simulink model "Ackerman Model For Simulation"  (R2020b)
settings: Solver=ode4  StartTime=0.0  StopTime=12  FixedStep=1e-5  RelTol=1e-3
InitFcn:
  | clc
  | clear
  | clc;
  | clear;
  | Ts=1e-5; %Sampling time
  | f=50; %Supply frequency
  | Rs=0.03553; %Stator resistance
  | Rr=0.02092; %Rotor resistance
  | Lls=0.000335; %Stator inductance
  | Llr=0.000335; %Rotor inductance
  | Lm=0.0151; %Mutual inductance
  | P=4; %Number of Poles
  | ts=(Lls+Lm)/Rs; % Stator time constant
  | Tr=(Llr+Lm)/Rr; % Rotor time constant
  | Ls=Lls+Lm;
  | Lr=Llr+Lm;
  | J=1.25; %Inertia
  | F=0.03914; %Friction factor
  | VDC=700;
  | sigma=1-(Lm^2/(Ls*Lr));
  | rs=Rs+Rr*(Lm/Lr)^2;
  | Kp=1498*sigma*Ls;
  | Ki=rs*1498;
  | dw=1.5;
  | l=2.5;
  | Kgear=2;
undefined symbols (not defined in the file): DiscIntNeverNeededParam
libraries: pid_lib x16, powerlib x13, powerlib_meascontrol x12, simulink_extras x2
(part 1 of 2)
settings Model: Creator=Mostafa  LastModifiedBy=Mostafa

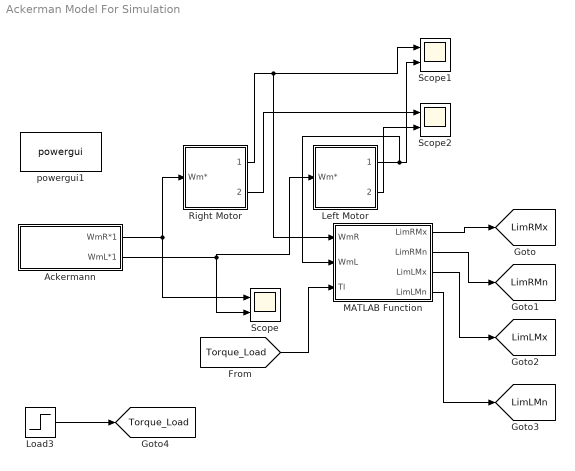
== system Ackerman Model For Simulation ==
  Ackermann : Subsystem
  Left Motor : Subsystem
  Load3 : Step  Time=0.5  After=200  SampleTime=Ts
  MATLAB Function : MATLAB Function  TreatAsAtomicUnit=on
  Right Motor : Subsystem
  Scope : Scope  NumInputPorts=2
  Scope1 : Scope  NumInputPorts=2
  Scope2 : Scope  NumInputPorts=2
  powergui1 : powerlib/powergui  Priority=1  SimulationMode=Continuous  SampleTime=1e-6  frequency=60  Iterations=50  frequencyindice=50  Pbase=100e6  ErrMax=1e-4  UnitsV=kV  UnitsW=MW  buscounter=0  FunctionMessages=off  echomessages=off  EnableUseOfTLC=off  CurrentSourceSwitches=off  DisableSnubberDevices=off  DisableRonSwitches=off  DisableVfSwitches=off  DisplayEquations=off  AutomaticDiscreteSolvers=off  SolverType=Tustin/Backward Euler (TBE)  Interpol=off  ExternalGateDelay=off  methode=off  Ts=100  x0status=blocks  SPID=on  SwTol=0  HookPort=off  NonlinearTolerance=1e-4  nMaxIteration=100  ContinueOnMaxIteration=off  RestoreLinks=warning  ResistiveCurrentMeasurement=off  Frange=[0:2:500]  Ylog=off  Xlog=on  ShowGrid=off  save=off  variable=ZData  structure=0  ZoomFFT=off  StartTime=0.0  cycles=1  DisplayStyle=1  fundamental=60  FreqAxis=off  MaxFrequency=1000  frequencyindicesteady=1  RmsSteady=1  display=off
  tag scope: LimLMn=global, LimLMx=global, LimRMn=global, LimRMx=global, Torque_Load=global
  wires:
  Ackermann/1(WmR*1) -> Right Motor/1(Wm*), Scope/1
  Ackermann/2(WmL*1) -> Scope/2, Left Motor/1(Wm*)
  Right Motor/1(SpeedR) -> MATLAB Function/1(WmR), Scope1/1
  MATLAB Function/1(LimRMx) -> [LimRMx]
  MATLAB Function/2(LimRMn) -> [LimRMn]
  MATLAB Function/3(LimLMx) -> [LimLMx]
  MATLAB Function/4(LimLMn) -> [LimLMn]
  [Torque_Load] -> MATLAB Function/3(Tl)
  Left Motor/1(SpeedL) -> MATLAB Function/2(WmL), Scope1/2
  Load3/1 -> [Torque_Load]
  Right Motor/2(TorqueR) -> Scope2/1
  Left Motor/2(TorqueL) -> Scope2/2

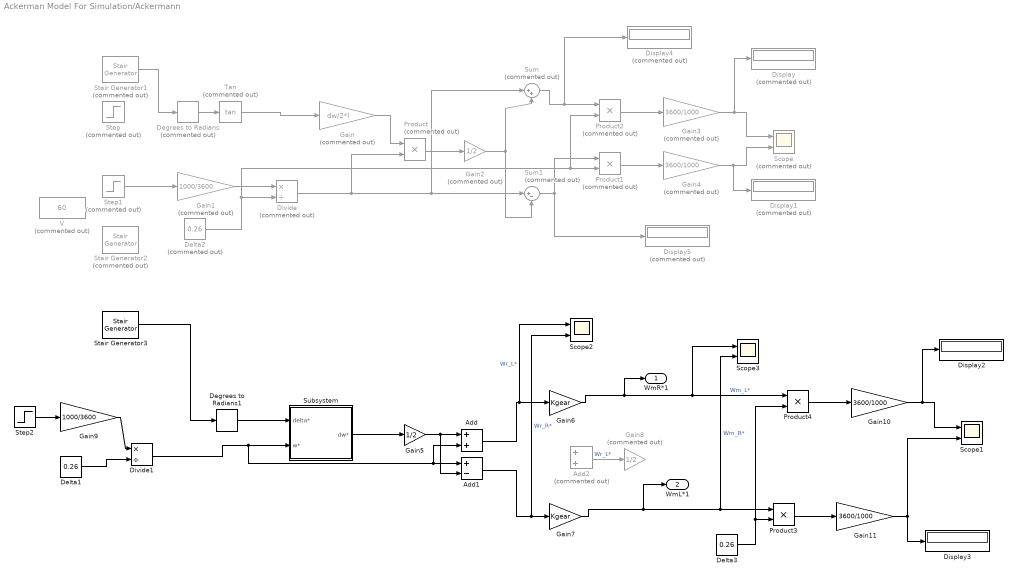
== system Ackerman Model For Simulation/Ackermann ==
  Add : Sum
  Add1 : Sum  Inputs=+-
  Add2 : Sum  Commented=on
  Degrees to Radians : simulink_extras/Transformations/Degrees to Radians  Commented=on
  Degrees to Radians1 : simulink_extras/Transformations/Degrees to Radians
  Delta1 : Constant  Value=0.26
  Delta2 : Constant  Commented=on  Value=0.26
  Delta3 : Constant  Value=0.26
  Display{,1,4..5} (4 alike) : Display  Commented=on
  Display2 : Display
  Display3 : Display
  Divide : Product  Commented=on  Inputs=*/
  Divide1 : Product  Inputs=*/
  Gain : Gain  Commented=on  Gain=dw/2*l
  Gain1 : Gain  Commented=on  Gain=1000/3600
  Gain10 : Gain  Gain=3600/1000
  Gain11 : Gain  Gain=3600/1000
  Gain2 : Gain  Commented=on  Gain=1/2
  Gain3 : Gain  Commented=on  Gain=3600/1000
  Gain4 : Gain  Commented=on  Gain=3600/1000
  Gain5 : Gain  Gain=1/2
  Gain6 : Gain  Gain=Kgear
  Gain7 : Gain  Gain=Kgear
  Gain8 : Gain  Commented=on  Gain=1/2
  Gain9 : Gain  Gain=1000/3600
  Product : Product  Commented=on
  Product1 : Product  Commented=on
  Product2 : Product  Commented=on
  Product3 : Product
  Product4 : Product
  Scope : Scope  Commented=on  NumInputPorts=2
  Scope1 : Scope  NumInputPorts=2
  Scope2 : Scope  NumInputPorts=2
  Scope3 : Scope  NumInputPorts=2
  Stair Generator1 : powerlib_meascontrol/Pulse & Signal Generators/Stair Generator  Commented=on  t="[0 4 6 8 10  ]"  e=[0 10 0 -10 0 ]  Ts=0
  Stair Generator2 : powerlib_meascontrol/Pulse & Signal Generators/Stair Generator  Commented=on  t=[0 3 5 7 9 10 ]  e=[0 50 100 -50 -100 0 ]  Ts=0
  Stair Generator3 : powerlib_meascontrol/Pulse & Signal Generators/Stair Generator  t="[0 4 6 8 10  ]"  e=[0 10 0 -10 0 ]  Ts=0
  Step : Step  Commented=on  Time=4  After=10  SampleTime=0
  Step1 : Step  Commented=on  Time=2.5  After=80  SampleTime=0
  Step2 : Step  Time=2.5  After=60  SampleTime=0
  Subsystem : Subsystem
  Sum : Sum  Commented=on  Inputs=|++
  Sum1 : Sum  Commented=on  Inputs=|+-
  Tan : Trigonometry  Commented=on  Operator=tan
  V : Constant  Commented=on  Value=60
  WmR*1 : Outport
  WmL*1 : Outport  Port=2
  wires:
  Degrees to Radians/1 -> Tan/1
  Tan/1 -> Gain/1
  Gain/1 -> Product/1
  Product/1 -> Gain2/1
  Gain2/1 -> Sum1/2, Sum/2
  Divide/1 -> Product/2, Sum/1, Sum1/1
  Gain1/1 -> Divide/1
  Sum1/1 -> Product1/1, Display5/1
  Delta2/1 -> Product2/2, Product1/2, Divide/2
  Product2/1 -> Gain3/1
  Product1/1 -> Gain4/1
  Gain4/1 -> Display1/1, Scope/2
  Gain3/1 -> Display/1, Scope/1
  Sum/1 -> Display4/1, Product2/1
  Stair Generator1/1 -> Degrees to Radians/1
  Step1/1 -> Gain1/1
  Gain7/1 -> WmL*1/1, Product3/1, Scope3/2  "Wm_R*"
  Gain11/1 -> Scope1/2, Display3/1
  Divide1/1 -> Add/2, Add1/1, Subsystem/2(w*)
  Gain9/1 -> Divide1/1
  Product4/1 -> Gain10/1
  Delta3/1 -> Product4/2, Product3/2
  Gain10/1 -> Scope1/1, Display2/1
  Step2/1 -> Gain9/1
  Add/1 -> Scope2/1, Gain6/1  "Wr_L*"
  Delta1/1 -> Divide1/2
  Degrees to Radians1/1 -> Subsystem/1(delta*)
  Product3/1 -> Gain11/1
  Add1/1 -> Scope2/2, Gain7/1  "Wr_R*"
  Gain6/1 -> WmR*1/1, Scope3/1, Product4/1  "Wm_L*"
  Gain5/1 -> Add1/2, Add/1
  Subsystem/1(dw*) -> Gain5/1
  Add2/1 -> Gain8/1  "Wr_L*"
  Stair Generator3/1 -> Degrees to Radians1/1

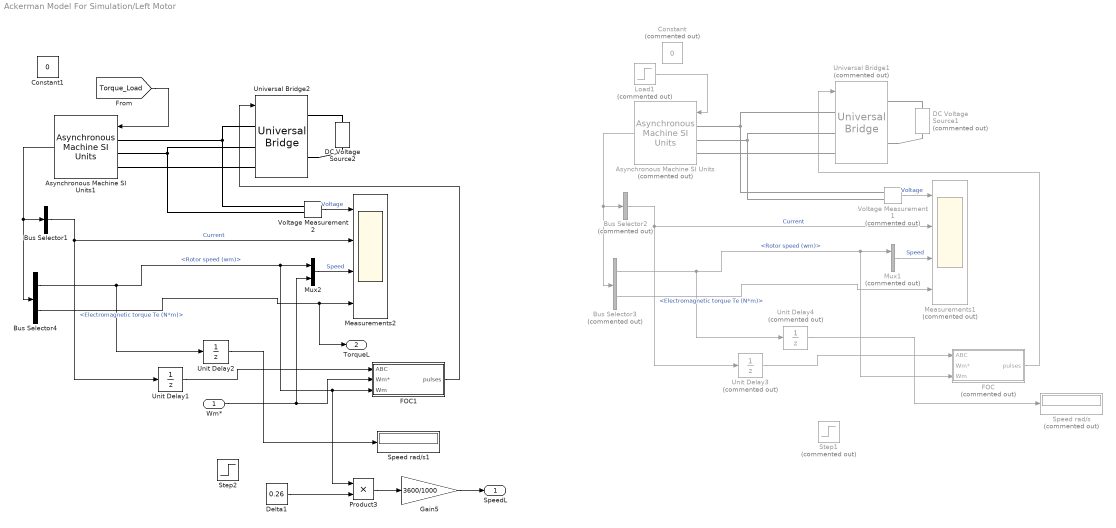
== system Ackerman Model For Simulation/Left Motor ==
  Wm* : Inport
  Asynchronous Machine SI Units : powerlib/Machines/Asynchronous Machine SI Units  Commented=on  RotorType=Squirrel-cage  PresetModel=No  MechanicalLoad=Torque Tm  ShowDetailedParameters=on  ReferenceFrame=Rotor  Units=SI  MeasurementBus=off  NominalParameters=[3*746 380 50]  Stator=[5.883 13.577e-3]  Rotor=[1.8993 13.577e-3]  Cage1=[0.4155 0.002066]  Cage2=[0.4168 0.0003495]  Lm=277e-3  Mechanical=[0.01 0.001 2]  PolePairs=2  InitialConditions=[1 0 0 0 0 0 0 0]  SimulateSaturation=off  Saturation=[14.03593122, 27.81365428, 53.79336849, 72.68890987, 97.98006896, 148.6815601, 215.7428561, 302.9841135, 428.7778367 ; 230, 322, 414, 460, 506, 552, 598, 644, 690]  LoadFlowParameters=1492000  TsPowergui=0  TsBlock=-1  IterativeModel=Trapezoidal non iterative  IterativeDiscreteModel=Trapezoidal non iterative  Pmec=1.492e+006
  Asynchronous Machine SI Units1 : powerlib/Machines/Asynchronous Machine SI Units  RotorType=Squirrel-cage  PresetModel="19:  100 HP (75KW)  400 V 50Hz 1484 RPM"  MechanicalLoad=Torque Tm  ShowDetailedParameters=on  ReferenceFrame=Rotor  Units=SI  MeasurementBus=off  NominalParameters=[7.5e+04 400 50]  Stator=[0.03552 0.000335]  Rotor=[0.02092 0.000335]  Cage1=[0.4155 0.002066]  Cage2=[0.4168 0.0003495]  Lm=0.0151  Mechanical=[1.25 0.03914 2]  PolePairs=2  InitialConditions=[1 0 0 0 0 0 0 0]  SimulateSaturation=off  Saturation=[14.03593122, 27.81365428, 53.79336849, 72.68890987, 97.98006896, 148.6815601, 215.7428561, 302.9841135, 428.7778367 ; 230, 322, 414, 460, 506, 552, 598, 644, 690]  LoadFlowParameters=1492000  TsPowergui=0  TsBlock=-1  IterativeModel=Trapezoidal non iterative  IterativeDiscreteModel=Trapezoidal non iterative  Pmec=1.492e+006
  Bus Selector1 : BusSelector  OutputSignals=Stator measurements.Stator current is_a (A),Stator measurements.Stator current is_b (A),Stator measurements.Stator current is_c (A)  OutputAsBus=on
  Bus Selector2 : BusSelector  Commented=on  OutputSignals=Stator measurements.Stator current is_a (A),Stator measurements.Stator current is_b (A),Stator measurements.Stator current is_c (A)  OutputAsBus=on
  Bus Selector3 : BusSelector  Commented=on  OutputSignals=Mechanical.Rotor speed (wm),Mechanical.Electromagnetic torque Te (N*m)
  Bus Selector4 : BusSelector  OutputSignals=Mechanical.Rotor speed (wm),Mechanical.Electromagnetic torque Te (N*m)
  Constant : Constant  Commented=on  Value=0
  Constant1 : Constant  Value=0
  DC Voltage Source1 : powerlib/Electrical Sources/DC Voltage Source  Commented=on  Amplitude=VDC  Measurements=None
  DC Voltage Source2 : powerlib/Electrical Sources/DC Voltage Source  Amplitude=VDC  Measurements=None
  Delta1 : Constant  Value=0.26
  FOC : Subsystem  Commented=on
  FOC1 : Subsystem
  Gain5 : Gain  Gain=3600/1000
  Load1 : Step  Commented=on  Time=0.5  After=8  SampleTime=Ts
  Measurements1 : Scope  Commented=on  NumInputPorts=4
  Measurements2 : Scope  NumInputPorts=4
  Mux1 : Mux  Commented=on  Inputs=2
  Mux2 : Mux  Inputs=2
  Product3 : Product
  Speed rad/s : Display  Commented=on
  Speed rad/s1 : Display
  Step1 : Step  Commented=on  Time=0.5  After=80  SampleTime=0
  Step2 : Step  Time=2.5  After=155  SampleTime=0
  Unit Delay1 : UnitDelay  SampleTime=-1  HasFrameUpgradeWarning=on
  Unit Delay2 : UnitDelay  SampleTime=-1  HasFrameUpgradeWarning=on
  Unit Delay3 : UnitDelay  Commented=on  SampleTime=-1  HasFrameUpgradeWarning=on
  Unit Delay4 : UnitDelay  Commented=on  SampleTime=-1  HasFrameUpgradeWarning=on
  Universal Bridge1 : powerlib/Power Electronics/Universal Bridge  Commented=on  Arms=3  SnubberResistance=1e5  SnubberCapacitance=inf  Device=IGBT / Diodes  Ron=1e-3  Lon=0  ForwardVoltages="[  0  0  ]"  ForwardVoltage=0  GTOparameters=[ 10e-6 , 20e-6 ]  IGBTparameters=[ 1e-6 , 2e-6 ]  Measurements=None  Measurements_2=None  converterType=Rectifier
  Universal Bridge2 : powerlib/Power Electronics/Universal Bridge  Arms=3  SnubberResistance=1e5  SnubberCapacitance=inf  Device=IGBT / Diodes  Ron=1e-3  Lon=0  ForwardVoltages="[  0  0  ]"  ForwardVoltage=0  GTOparameters=[ 10e-6 , 20e-6 ]  IGBTparameters=[ 1e-6 , 2e-6 ]  Measurements=None  Measurements_2=None  converterType=Rectifier
  Voltage Measurement1 : powerlib/Measurements/Voltage Measurement  Commented=on  PhasorSimulation=off  OutputType=Complex  PSBequivalent=0
  Voltage Measurement2 : powerlib/Measurements/Voltage Measurement  PhasorSimulation=off  OutputType=Complex  PSBequivalent=0
  SpeedL : Outport
  TorqueL : Outport  Port=2
  wires:
  Wm*/1 -> FOC1/2(Wm*), Mux2/2
  Voltage Measurement2/1 -> Measurements2/1  "Voltage"
  Asynchronous Machine SI Units1/1 -> Bus Selector1/1, Bus Selector4/1
  Bus Selector1/1 -> Measurements2/2, Unit Delay1/1  "Current"
  Bus Selector4/1 -> Unit Delay2/1, Mux2/1, Product3/1, FOC1/3(Wm)  "<Rotor speed (wm)>"
  Unit Delay2/1 -> Speed rad/s1/1
  Bus Selector4/2 -> TorqueL/1, Measurements2/4  "<Electromagnetic torque Te (N*m)>"
  Mux2/1 -> Measurements2/3  "Speed"
  Unit Delay1/1 -> FOC1/1(ABC)
  FOC1/1(pulses) -> Universal Bridge2/1
  Load1/1 -> Asynchronous Machine SI Units/1
  Unit Delay4/1 -> Speed rad/s/1
  Unit Delay3/1 -> FOC/1(ABC)
  Bus Selector3/1 -> Unit Delay4/1, Mux1/1, FOC/3(Wm)  "<Rotor speed (wm)>"
  Voltage Measurement1/1 -> Measurements1/1  "Voltage"
  Mux1/1 -> Measurements1/3  "Speed"
  Asynchronous Machine SI Units/1 -> Bus Selector2/1, Bus Selector3/1
  Bus Selector2/1 -> Measurements1/2, Unit Delay3/1  "Current"
  Bus Selector3/2 -> Measurements1/4  "<Electromagnetic torque Te (N*m)>"
  FOC/1(pulses) -> Universal Bridge1/1
  [Torque_Load] -> Asynchronous Machine SI Units1/1
  Delta1/1 -> Product3/2
  Product3/1 -> Gain5/1
  Gain5/1 -> SpeedL/1
  connections:
  Universal Bridge2/RConn2 -- DC Voltage Source2/LConn1
  Universal Bridge2/RConn1 -- DC Voltage Source2/RConn1
  Asynchronous Machine SI Units1/LConn3 -- Universal Bridge2/LConn3
  Voltage Measurement2/LConn2 -- Universal Bridge2/LConn2 -- Asynchronous Machine SI Units1/LConn2
  Universal Bridge2/LConn1 -- Voltage Measurement2/LConn1 -- Asynchronous Machine SI Units1/LConn1
  Asynchronous Machine SI Units/LConn3 -- Universal Bridge1/LConn3
  Universal Bridge1/RConn1 -- DC Voltage Source1/RConn1
  Universal Bridge1/RConn2 -- DC Voltage Source1/LConn1
  Asynchronous Machine SI Units/LConn2 -- Universal Bridge1/LConn2 -- Voltage Measurement1/LConn2
  Asynchronous Machine SI Units/LConn1 -- Universal Bridge1/LConn1 -- Voltage Measurement1/LConn1

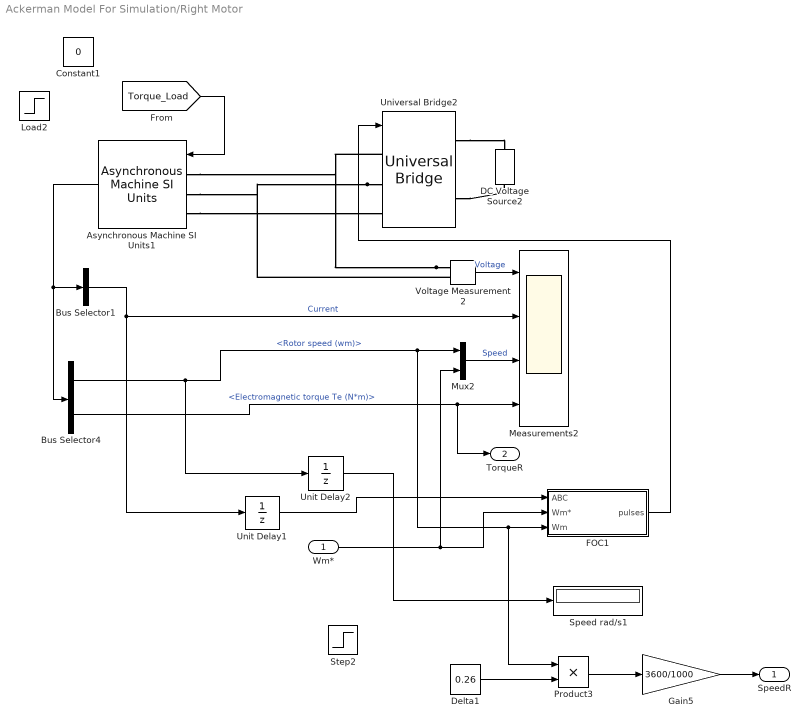
== system Ackerman Model For Simulation/Right Motor ==
  Wm* : Inport
  Asynchronous Machine SI Units1 : powerlib/Machines/Asynchronous Machine SI Units  RotorType=Squirrel-cage  PresetModel="19:  100 HP (75KW)  400 V 50Hz 1484 RPM"  MechanicalLoad=Torque Tm  ShowDetailedParameters=on  ReferenceFrame=Rotor  Units=SI  MeasurementBus=off  NominalParameters=[7.5e+04 400 50]  Stator=[0.03552 0.000335]  Rotor=[0.02092 0.000335]  Cage1=[0.4155 0.002066]  Cage2=[0.4168 0.0003495]  Lm=0.0151  Mechanical=[1.25 0.03914 2]  PolePairs=2  InitialConditions=[1 0 0 0 0 0 0 0]  SimulateSaturation=off  Saturation=[14.03593122, 27.81365428, 53.79336849, 72.68890987, 97.98006896, 148.6815601, 215.7428561, 302.9841135, 428.7778367 ; 230, 322, 414, 460, 506, 552, 598, 644, 690]  LoadFlowParameters=1492000  TsPowergui=0  TsBlock=-1  IterativeModel=Trapezoidal non iterative  IterativeDiscreteModel=Trapezoidal non iterative  Pmec=1.492e+006
  Bus Selector1 : BusSelector  OutputSignals=Stator measurements.Stator current is_a (A),Stator measurements.Stator current is_b (A),Stator measurements.Stator current is_c (A)  OutputAsBus=on
  Bus Selector4 : BusSelector  OutputSignals=Mechanical.Rotor speed (wm),Mechanical.Electromagnetic torque Te (N*m)
  Constant1 : Constant  Value=0
  DC Voltage Source2 : powerlib/Electrical Sources/DC Voltage Source  Amplitude=VDC  Measurements=None
  Delta1 : Constant  Value=0.26
  FOC1 : Subsystem
  Gain5 : Gain  Gain=3600/1000
  Load2 : Step  Time=0.5  After=3  SampleTime=Ts
  Measurements2 : Scope  NumInputPorts=4
  Mux2 : Mux  Inputs=2
  Product3 : Product
  Speed rad/s1 : Display
  Step2 : Step  Time=2.5  After=155  SampleTime=0
  Unit Delay1 : UnitDelay  SampleTime=-1  HasFrameUpgradeWarning=on
  Unit Delay2 : UnitDelay  SampleTime=-1  HasFrameUpgradeWarning=on
  Universal Bridge2 : powerlib/Power Electronics/Universal Bridge  Arms=3  SnubberResistance=1e5  SnubberCapacitance=inf  Device=IGBT / Diodes  Ron=1e-3  Lon=0  ForwardVoltages="[  0  0  ]"  ForwardVoltage=0  GTOparameters=[ 10e-6 , 20e-6 ]  IGBTparameters=[ 1e-6 , 2e-6 ]  Measurements=None  Measurements_2=None  converterType=Rectifier
  Voltage Measurement2 : powerlib/Measurements/Voltage Measurement  PhasorSimulation=off  OutputType=Complex  PSBequivalent=0
  SpeedR : Outport
  TorqueR : Outport  Port=2
  wires:
  FOC1/1(pulses) -> Universal Bridge2/1
  Unit Delay1/1 -> FOC1/1(ABC)
  Mux2/1 -> Measurements2/3  "Speed"
  Bus Selector4/2 -> TorqueR/1, Measurements2/4  "<Electromagnetic torque Te (N*m)>"
  Unit Delay2/1 -> Speed rad/s1/1
  Bus Selector4/1 -> Product3/1, FOC1/3(Wm), Mux2/1, Unit Delay2/1  "<Rotor speed (wm)>"
  Bus Selector1/1 -> Unit Delay1/1, Measurements2/2  "Current"
  Asynchronous Machine SI Units1/1 -> Bus Selector4/1, Bus Selector1/1
  Voltage Measurement2/1 -> Measurements2/1  "Voltage"
  Wm*/1 -> Mux2/2, FOC1/2(Wm*)
  [Torque_Load] -> Asynchronous Machine SI Units1/1
  Delta1/1 -> Product3/2
  Gain5/1 -> SpeedR/1
  Product3/1 -> Gain5/1
  connections:
  Voltage Measurement2/LConn1 -- Universal Bridge2/LConn1 -- Asynchronous Machine SI Units1/LConn1
  Universal Bridge2/LConn2 -- Voltage Measurement2/LConn2 -- Asynchronous Machine SI Units1/LConn2
  Asynchronous Machine SI Units1/LConn3 -- Universal Bridge2/LConn3
  Universal Bridge2/RConn1 -- DC Voltage Source2/RConn1
  Universal Bridge2/RConn2 -- DC Voltage Source2/LConn1

== system Ackerman Model For Simulation/Ackermann/Subsystem ==
  delta* : Inport
  w* : Inport  Port=2
  Constant : Constant  Value=dw
  Constant1 : Constant  Value=l
  Divide : Product  Inputs=**
  Divide1 : Product  Inputs=*/
  Divide2 : Product  Inputs=**
  Tan : Trigonometry  Operator=tan
  dw* : Outport
  wires:
  delta*/1 -> Tan/1
  Tan/1 -> Divide/1
  Constant/1 -> Divide/2
  Divide/1 -> Divide1/1
  Constant1/1 -> Divide1/2
  Divide1/1 -> Divide2/1
  w*/1 -> Divide2/2
  Divide2/1 -> dw*/1

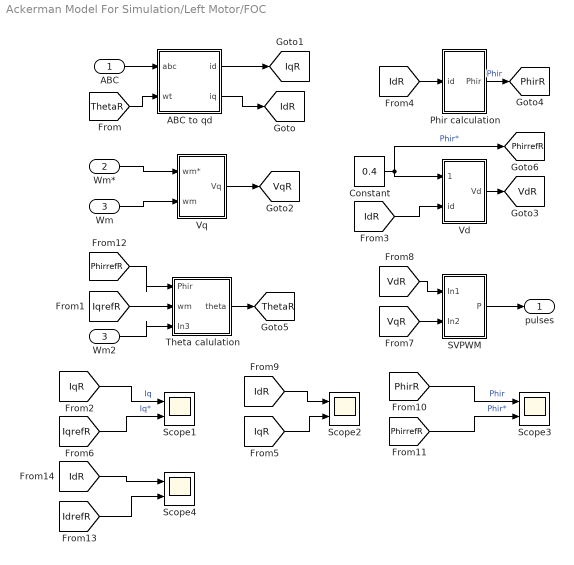
== system Ackerman Model For Simulation/Left Motor/FOC ==
  ABC : Inport
  Wm* : Inport  Port=2
  Wm : Inport  Port=3
  ABC to qd : Subsystem
  Constant : Constant  Value=0.4
  Phir calculation : Subsystem
  SVPWM : Subsystem
  Scope{1..4} (4 alike) : Scope  NumInputPorts=2
  Theta calulation : Subsystem
  Vd : Subsystem
  Vq : Subsystem
  Wm2 : InportShadow  Port=3
  pulses : Outport
  tag scope: IdR=global, IqR=global, PhirR=global, PhirrefR=global, ThetaR=global, VdR=global, VqR=global
  wires:
  [IdrefR] -> Scope4/2
  [IdR] -> Scope4/1
  [PhirrefR] -> Theta calulation/1(Phir)
  [PhirR] -> Scope3/1  "Phir"
  [PhirrefR] -> Scope3/2  "Phir*"
  [IdR] -> Scope2/1
  [IqR] -> Scope2/2
  [IqrefR] -> Scope1/2  "Iq*"
  [IqR] -> Scope1/1  "Iq"
  [IqrefR] -> Theta calulation/2(wm)
  Vd/1(Vd) -> [VdR]
  [IdR] -> Vd/2(id)
  Constant/1 -> [PhirrefR], Vd/1(Phir*)  "Phir*"
  Theta calulation/1(theta) -> [ThetaR]
  Wm2/1 -> Theta calulation/3(In3)
  SVPWM/1(P) -> pulses/1
  [VqR] -> SVPWM/2(In2)
  [VdR] -> SVPWM/1(In1)
  Phir calculation/1(Phir) -> [PhirR]  "Phir"
  [IdR] -> Phir calculation/1(id)
  ABC to qd/2(iq) -> [IdR]
  ABC to qd/1(id) -> [IqR]
  [ThetaR] -> ABC to qd/2(wt)
  ABC/1 -> ABC to qd/1(abc)
  Vq/1(Vq) -> [VqR]
  Wm/1 -> Vq/2(wm)
  Wm*/1 -> Vq/1(wm*)

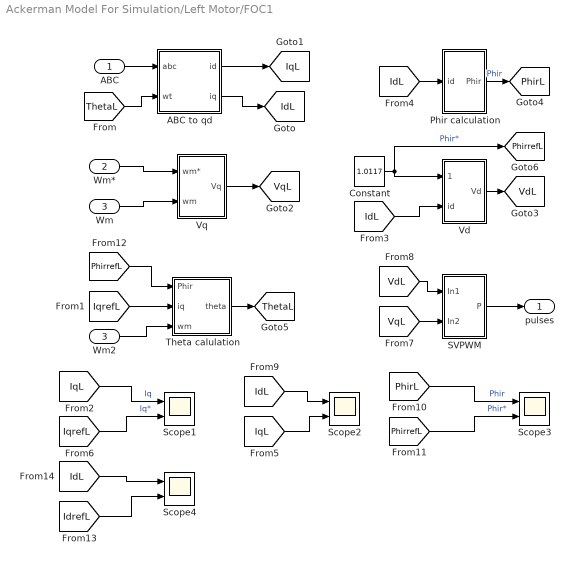
== system Ackerman Model For Simulation/Left Motor/FOC1 ==
  ABC : Inport
  Wm* : Inport  Port=2
  Wm : Inport  Port=3
  ABC to qd : Subsystem
  Constant : Constant  Value=1.0117
  Phir calculation : Subsystem
  SVPWM : Subsystem
  Scope{1..4} (4 alike) : Scope  NumInputPorts=2
  Theta calulation : Subsystem
  Vd : Subsystem
  Vq : Subsystem
  Wm2 : InportShadow  Port=3
  pulses : Outport
  tag scope: IdL=global, IqL=global, PhirL=global, PhirrefL=global, ThetaL=global, VdL=global, VqL=global
  wires:
  [IqrefL] -> Theta calulation/2(iq)
  [PhirrefL] -> Theta calulation/1(Phir)
  [IdrefL] -> Scope4/2
  [IdL] -> Scope4/1
  [PhirL] -> Scope3/1  "Phir"
  [PhirrefL] -> Scope3/2  "Phir*"
  [IdL] -> Scope2/1
  [IqL] -> Scope2/2
  [IqrefL] -> Scope1/2  "Iq*"
  [IqL] -> Scope1/1  "Iq"
  Vd/1(Vd) -> [VdL]
  [IdL] -> Vd/2(id)
  Constant/1 -> [PhirrefL], Vd/1(Phir*)  "Phir*"
  Theta calulation/1(theta) -> [ThetaL]
  Wm2/1 -> Theta calulation/3(wm)
  SVPWM/1(P) -> pulses/1
  [VqL] -> SVPWM/2(In2)
  [VdL] -> SVPWM/1(In1)
  Phir calculation/1(Phir) -> [PhirL]  "Phir"
  [IdL] -> Phir calculation/1(id)
  ABC to qd/2(iq) -> [IdL]
  ABC to qd/1(id) -> [IqL]
  [ThetaL] -> ABC to qd/2(wt)
  ABC/1 -> ABC to qd/1(abc)
  Vq/1(Vq) -> [VqL]
  Wm/1 -> Vq/2(wm)
  Wm*/1 -> Vq/1(wm*)

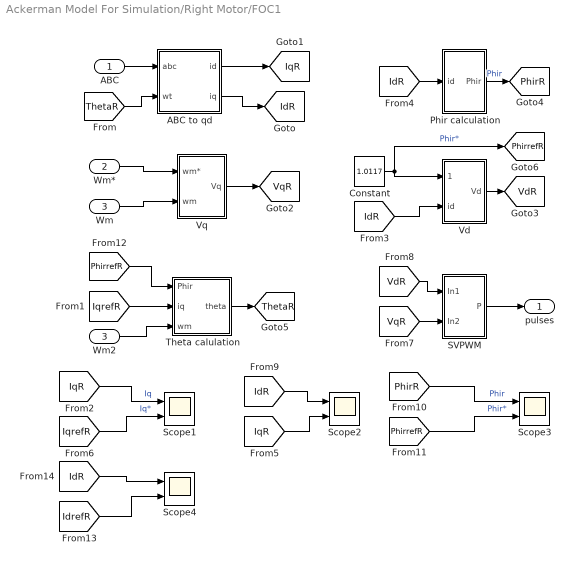
== system Ackerman Model For Simulation/Right Motor/FOC1 ==
  ABC : Inport
  Wm* : Inport  Port=2
  Wm : Inport  Port=3
  ABC to qd : Subsystem
  Constant : Constant  Value=1.0117
  Phir calculation : Subsystem
  SVPWM : Subsystem
  Scope{1..4} (4 alike) : Scope  NumInputPorts=2
  Theta calulation : Subsystem
  Vd : Subsystem
  Vq : Subsystem
  Wm2 : InportShadow  Port=3
  pulses : Outport
  tag scope: IdR=global, IqR=global, PhirR=global, PhirrefR=global, ThetaR=global, VdR=global, VqR=global
  wires:
  Wm*/1 -> Vq/1(wm*)
  Wm/1 -> Vq/2(wm)
  Vq/1(Vq) -> [VqR]
  ABC/1 -> ABC to qd/1(abc)
  [ThetaR] -> ABC to qd/2(wt)
  ABC to qd/1(id) -> [IqR]
  ABC to qd/2(iq) -> [IdR]
  [IdR] -> Phir calculation/1(id)
  Phir calculation/1(Phir) -> [PhirR]  "Phir"
  [VdR] -> SVPWM/1(In1)
  [VqR] -> SVPWM/2(In2)
  SVPWM/1(P) -> pulses/1
  Wm2/1 -> Theta calulation/3(wm)
  Theta calulation/1(theta) -> [ThetaR]
  Constant/1 -> Vd/1(Phir*), [PhirrefR]  "Phir*"
  [IdR] -> Vd/2(id)
  Vd/1(Vd) -> [VdR]
  [IqR] -> Scope1/1  "Iq"
  [IqrefR] -> Scope1/2  "Iq*"
  [IqR] -> Scope2/2
  [IdR] -> Scope2/1
  [PhirrefR] -> Scope3/2  "Phir*"
  [PhirR] -> Scope3/1  "Phir"
  [IdR] -> Scope4/1
  [IdrefR] -> Scope4/2
  [PhirrefR] -> Theta calulation/1(Phir)
  [IqrefR] -> Theta calulation/2(iq)

== system Ackerman Model For Simulation/Left Motor/FOC/ABC to qd ==
  abc : Inport
  wt : Inport  Port=2
  Demux : Demux  Outputs=3
  Terminator : Terminator
  Unit Delay : UnitDelay  SampleTime=-1  HasFrameUpgradeWarning=on
  Unit Delay1 : UnitDelay  SampleTime=-1  HasFrameUpgradeWarning=on
  abc to dq0 : powerlib_meascontrol/Transformations/abc to dq0  Alignment=90 degrees behind phase A axis
  id : Outport
  iq : Outport  Port=2
  wires:
  abc/1 -> abc to dq0/1
  Unit Delay1/1 -> id/1
  wt/1 -> abc to dq0/2
  Unit Delay/1 -> iq/1
  Demux/2 -> Unit Delay1/1
  abc to dq0/1 -> Demux/1
  Demux/3 -> Terminator/1
  Demux/1 -> Unit Delay/1

== system Ackerman Model For Simulation/Left Motor/FOC/Phir calculation ==
  id : Inport
  Transfer Fcn : TransferFcn  Numerator=[Lm]  Denominator=[Tr 1]
  Phir : Outport
  wires:
  id/1 -> Transfer Fcn/1
  Transfer Fcn/1 -> Phir/1

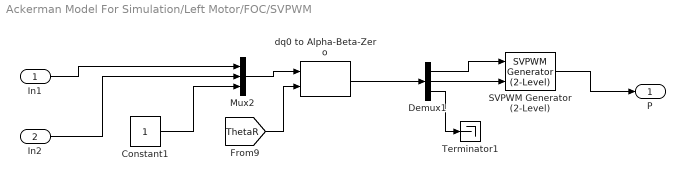
== system Ackerman Model For Simulation/Left Motor/FOC/SVPWM ==
  In1 : Inport
  In2 : Inport  Port=2
  Constant1 : Constant
  Demux1 : Demux  Outputs=3
  Mux2 : Mux  Inputs=3
  SVPWM Generator (2-Level) : powerlib_meascontrol/Pulse & Signal Generators/SVPWM Generator (2-Level)  InputType=alpha-beta components  SwitchingPattern=Pattern #1  Fc=5000  ParUref=[0.8 -30 50]  Ts=0
      settings: SourceProductBaseCode=PS
  Terminator1 : Terminator
  dq0 to Alpha-Beta-Zero : powerlib_meascontrol/Transformations/dq0 to Alpha-Beta-Zero  Alignment=90 degrees behind phase A axis
      settings: SourceProductBaseCode=PS
  P : Outport
  wires:
  Demux1/1 -> SVPWM Generator (2-Level)/1
  Constant1/1 -> Mux2/3
  dq0 to Alpha-Beta-Zero/1 -> Demux1/1
  [ThetaR] -> dq0 to Alpha-Beta-Zero/2
  In2/1 -> Mux2/2
  SVPWM Generator (2-Level)/1 -> P/1
  In1/1 -> Mux2/1
  Mux2/1 -> dq0 to Alpha-Beta-Zero/1
  Demux1/3 -> Terminator1/1
  Demux1/2 -> SVPWM Generator (2-Level)/2

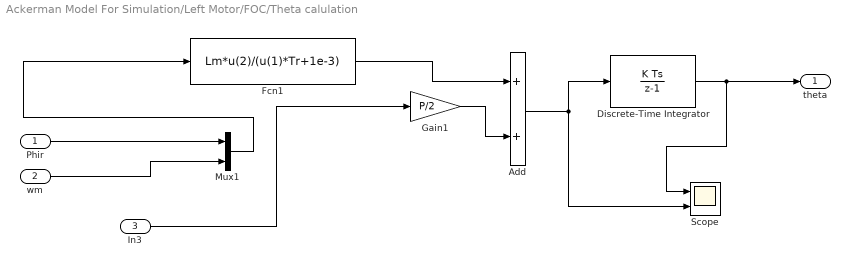
== system Ackerman Model For Simulation/Left Motor/FOC/Theta calulation ==
  Phir : Inport
  wm : Inport  Port=2
  In3 : Inport  Port=3
  Add : Sum
  Discrete-Time Integrator : DiscreteIntegrator  SampleTime=Ts  ICPrevOutput=DiscIntNeverNeededParam  ICPrevScaledInput=DiscIntNeverNeededParam
  Fcn1 : Fcn  Expr=Lm*u(2)/(u(1)*Tr+1e-3)
  Gain1 : Gain  Gain=P/2
  Mux1 : Mux  Inputs=2
  Scope : Scope  NumInputPorts=2
  theta : Outport
  wires:
  Discrete-Time Integrator/1 -> theta/1, Scope/1
  wm/1 -> Mux1/2
  In3/1 -> Gain1/1
  Add/1 -> Discrete-Time Integrator/1, Scope/2
  Mux1/1 -> Fcn1/1
  Fcn1/1 -> Add/1
  Phir/1 -> Mux1/1
  Gain1/1 -> Add/2

== system Ackerman Model For Simulation/Left Motor/FOC/Vd ==
  Phir* : Inport
  id : Inport  Port=2
  Current PI : pid_lib/PID Controller  Controller=PI  Form=Parallel  TimeDomain=Discrete-time  UseExternalTs=off  SampleTime=Ts  IntegratorMethod=Forward Euler  FilterMethod=Forward Euler  ControllerParametersSource=internal  P=39.67  I=11365  D=0  UseFilter=on  N=100  TunerSelectOption=Transfer Function Based (PID Tuner App)  InitialConditionSource=internal  InitialConditionForIntegrator=0  InitialConditionForFilter=0  DifferentiatorICPrevScaledInput=0  ExternalReset=none  TrackingMode=off  Kt=1  LimitOutput=on  SatLimitsSource=internal  UpperSaturationLimit=VDC  LowerSaturationLimit=-VDC/2  LinearizeAsGain=off  AntiWindupMode=clamping  Kb=1  POutMin=[]  POutMax=[]  IOutMin=[]  IOutMax=[]  DOutMin=[]  DOutMax=[]  NOutMin=[]  NOutMax=[]  SumOutMin=[]  SumOutMax=[]  SaturationOutMin=[]  SaturationOutMax=[]  PParamMin=[]  PParamMax=[]  IParamMin=[]  IParamMax=[]  DParamMin=[]  DParamMax=[]  NParamMin=[]  NParamMax=[]  KbParamMin=[]  KbParamMax=[]  KtParamMin=[]  KtParamMax=[]  KbOutMin=[]  KbOutMax=[]  KtOutMin=[]  KtOutMax=[]  IntegratorOutMin=[]  IntegratorOutMax=[]  FilterOutMin=[]  FilterOutMax=[]  SumI1OutMin=[]  SumI1OutMax=[]  SumI2OutMin=[]  SumI2OutMax=[]  SumI3OutMin=[]  SumI3OutMax=[]  SumI4OutMin=[]  SumI4OutMax=[]  SumDOutMin=[]  SumDOutMax=[]  DifferentiatorOutMin=[]  DifferentiatorOutMax=[]  FilterDiffOutCoefMin=[]  FilterDiffOutCoefMax=[]  ReciprocalOutMin=[]  ReciprocalOutMax=[]  SumDenOutMin=[]  SumDenOutMax=[]  SumNumOutMin=[]  SumNumOutMax=[]  DivideOutMin=[]  DivideOutMax=[]  UdiffTsProdOutMin=[]  UdiffTsProdOutMax=[]  NTsProdOutMin=[]  NTsProdOutMax=[]  UintegralTsProdOutMin=[]  UintegralTsProdOutMax=[]  UngainTsProdOutMin=[]  UngainTsProdOutMax=[]  IntegratorContinuousStateAttributes=''  IntegratorStateMustResolveToSignalObject=off  IntegratorRTWStateStorageClass=Auto  FilterContinuousStateAttributes=''  FilterStateMustResolveToSignalObject=off  FilterRTWStateStorageClass=Auto  ParallelPVariant=InternalParameters  IdealPVariant=Disabled  IVariant=InternalParameters  DVariant=Disabled  IntegratorVariant=Discrete  SatVariant=Enabled  AWVariant=DiscClampingParallel  PCopyVariant=Disabled  TRVariant=Disabled  FdbkBlocksVariant=Forward  IdealPFdbkVariant=Disabled  SatFdbkVariant=Disabled  DerivativeFilterVariant=Disabled  NVariant=Disabled  NCopyVariant=Disabled_SignalSpec  FilterICVariant=Disabled  IntegratorICVariant=InternalICs  ExternalResetVariant=Disabled  TRSumVariant=Passthrough  SumFdbkVariant=Disabled  SumVariant=Sum_PI  TsampFilterVariant=InternalTs  TsampNgainVariant=Passthrough  TsampIntegralVariant=Passthrough  ExternalSaturationOutDataTypeStr=Inherit: Same as second input
  Gain : Gain  Gain=1/Lm
  Scope : Scope
  Sum2 : Sum  Inputs=|+-
  Vd : Outport
  tag scope: IdrefR=global
  wires:
  Current PI/1 -> Vd/1
  Sum2/1 -> Current PI/1
  id/1 -> Sum2/2
  Phir*/1 -> Gain/1
  Gain/1 -> Sum2/1, Scope/1, [IdrefR]

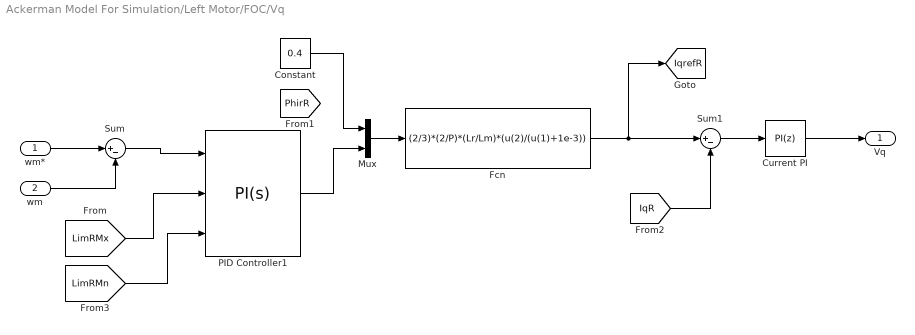
== system Ackerman Model For Simulation/Left Motor/FOC/Vq ==
  wm* : Inport
  wm : Inport  Port=2
  Constant : Constant  Value=0.4
  Current PI : pid_lib/PID Controller  Controller=PI  Form=Parallel  TimeDomain=Discrete-time  UseExternalTs=off  SampleTime=Ts  IntegratorMethod=Forward Euler  FilterMethod=Forward Euler  ControllerParametersSource=internal  P=39.67  I=11365  D=0  UseFilter=on  N=100  TunerSelectOption=Transfer Function Based (PID Tuner App)  InitialConditionSource=internal  InitialConditionForIntegrator=0  InitialConditionForFilter=0  DifferentiatorICPrevScaledInput=0  ExternalReset=none  TrackingMode=off  Kt=1  LimitOutput=on  SatLimitsSource=internal  UpperSaturationLimit=VDC/2  LowerSaturationLimit=-VDC/2  LinearizeAsGain=off  AntiWindupMode=clamping  Kb=1  POutMin=[]  POutMax=[]  IOutMin=[]  IOutMax=[]  DOutMin=[]  DOutMax=[]  NOutMin=[]  NOutMax=[]  SumOutMin=[]  SumOutMax=[]  SaturationOutMin=[]  SaturationOutMax=[]  PParamMin=[]  PParamMax=[]  IParamMin=[]  IParamMax=[]  DParamMin=[]  DParamMax=[]  NParamMin=[]  NParamMax=[]  KbParamMin=[]  KbParamMax=[]  KtParamMin=[]  KtParamMax=[]  KbOutMin=[]  KbOutMax=[]  KtOutMin=[]  KtOutMax=[]  IntegratorOutMin=[]  IntegratorOutMax=[]  FilterOutMin=[]  FilterOutMax=[]  SumI1OutMin=[]  SumI1OutMax=[]  SumI2OutMin=[]  SumI2OutMax=[]  SumI3OutMin=[]  SumI3OutMax=[]  SumI4OutMin=[]  SumI4OutMax=[]  SumDOutMin=[]  SumDOutMax=[]  DifferentiatorOutMin=[]  DifferentiatorOutMax=[]  FilterDiffOutCoefMin=[]  FilterDiffOutCoefMax=[]  ReciprocalOutMin=[]  ReciprocalOutMax=[]  SumDenOutMin=[]  SumDenOutMax=[]  SumNumOutMin=[]  SumNumOutMax=[]  DivideOutMin=[]  DivideOutMax=[]  UdiffTsProdOutMin=[]  UdiffTsProdOutMax=[]  NTsProdOutMin=[]  NTsProdOutMax=[]  UintegralTsProdOutMin=[]  UintegralTsProdOutMax=[]  UngainTsProdOutMin=[]  UngainTsProdOutMax=[]  IntegratorContinuousStateAttributes=''  IntegratorStateMustResolveToSignalObject=off  IntegratorRTWStateStorageClass=Auto  FilterContinuousStateAttributes=''  FilterStateMustResolveToSignalObject=off  FilterRTWStateStorageClass=Auto  ParallelPVariant=InternalParameters  IdealPVariant=Disabled  IVariant=InternalParameters  DVariant=Disabled  IntegratorVariant=Discrete  SatVariant=Enabled  AWVariant=DiscClampingParallel  PCopyVariant=Disabled  TRVariant=Disabled  FdbkBlocksVariant=Forward  IdealPFdbkVariant=Disabled  SatFdbkVariant=Disabled  DerivativeFilterVariant=Disabled  NVariant=Disabled  NCopyVariant=Disabled_SignalSpec  FilterICVariant=Disabled  IntegratorICVariant=InternalICs  ExternalResetVariant=Disabled  TRSumVariant=Passthrough  SumFdbkVariant=Disabled  SumVariant=Sum_PI  TsampFilterVariant=InternalTs  TsampNgainVariant=Passthrough  TsampIntegralVariant=Passthrough  ExternalSaturationOutDataTypeStr=Inherit: Same as second input
  Fcn : Fcn  Expr=(2/3)*(2/P)*(Lr/Lm)*(u(2)/(u(1)+1e-3))
  Mux : Mux  Inputs=2
  PID Controller1 : pid_lib/PID Controller  Controller=PI  Form=Parallel  TimeDomain=Continuous-time  UseExternalTs=off  SampleTime=-1  IntegratorMethod=Forward Euler  FilterMethod=Forward Euler  ControllerParametersSource=internal  P=3  I=16  D=0  UseFilter=on  N=100  TunerSelectOption=Transfer Function Based (PID Tuner App)  InitialConditionSource=internal  InitialConditionForIntegrator=0  InitialConditionForFilter=0  DifferentiatorICPrevScaledInput=0  ExternalReset=none  TrackingMode=off  Kt=1  LimitOutput=on  SatLimitsSource=external  UpperSaturationLimit=15  LowerSaturationLimit=-15  LinearizeAsGain=off  AntiWindupMode=clamping  Kb=1  POutMin=[]  POutMax=[]  IOutMin=[]  IOutMax=[]  DOutMin=[]  DOutMax=[]  NOutMin=[]  NOutMax=[]  SumOutMin=[]  SumOutMax=[]  SaturationOutMin=[]  SaturationOutMax=[]  PParamMin=[]  PParamMax=[]  IParamMin=[]  IParamMax=[]  DParamMin=[]  DParamMax=[]  NParamMin=[]  NParamMax=[]  KbParamMin=[]  KbParamMax=[]  KtParamMin=[]  KtParamMax=[]  KbOutMin=[]  KbOutMax=[]  KtOutMin=[]  KtOutMax=[]  IntegratorOutMin=[]  IntegratorOutMax=[]  FilterOutMin=[]  FilterOutMax=[]  SumI1OutMin=[]  SumI1OutMax=[]  SumI2OutMin=[]  SumI2OutMax=[]  SumI3OutMin=[]  SumI3OutMax=[]  SumI4OutMin=[]  SumI4OutMax=[]  SumDOutMin=[]  SumDOutMax=[]  DifferentiatorOutMin=[]  DifferentiatorOutMax=[]  FilterDiffOutCoefMin=[]  FilterDiffOutCoefMax=[]  ReciprocalOutMin=[]  ReciprocalOutMax=[]  SumDenOutMin=[]  SumDenOutMax=[]  SumNumOutMin=[]  SumNumOutMax=[]  DivideOutMin=[]  DivideOutMax=[]  UdiffTsProdOutMin=[]  UdiffTsProdOutMax=[]  NTsProdOutMin=[]  NTsProdOutMax=[]  UintegralTsProdOutMin=[]  UintegralTsProdOutMax=[]  UngainTsProdOutMin=[]  UngainTsProdOutMax=[]  IntegratorContinuousStateAttributes=''  IntegratorStateMustResolveToSignalObject=off  IntegratorRTWStateStorageClass=Auto  FilterContinuousStateAttributes=''  FilterStateMustResolveToSignalObject=off  FilterRTWStateStorageClass=Auto  ParallelPVariant=InternalParameters  IdealPVariant=Disabled  IVariant=InternalParameters  DVariant=Disabled  IntegratorVariant=Continuous  SatVariant=External  AWVariant=ContClampingParallel  PCopyVariant=Disabled  TRVariant=Disabled  FdbkBlocksVariant=Forward  IdealPFdbkVariant=Disabled  SatFdbkVariant=Disabled  DerivativeFilterVariant=Disabled  NVariant=Disabled  NCopyVariant=Disabled_SignalSpec  FilterICVariant=Disabled  IntegratorICVariant=InternalICs  ExternalResetVariant=Disabled  TRSumVariant=Passthrough  SumFdbkVariant=Disabled  SumVariant=Sum_PI  TsampFilterVariant=InternalTs  TsampNgainVariant=Passthrough  TsampIntegralVariant=Passthrough  ExternalSaturationOutDataTypeStr=Inherit: Same as second input
  Sum : Sum  Inputs=|+-
  Sum1 : Sum  Inputs=|+-
  Vq : Outport
  tag scope: IqrefR=global
  wires:
  [LimRMn] -> PID Controller1/3
  [LimRMx] -> PID Controller1/2
  PID Controller1/1 -> Mux/2
  Sum/1 -> PID Controller1/1
  Constant/1 -> Mux/1
  Current PI/1 -> Vq/1
  Sum1/1 -> Current PI/1
  Fcn/1 -> [IqrefR], Sum1/1
  [IqR] -> Sum1/2
  wm*/1 -> Sum/1
  Mux/1 -> Fcn/1
  wm/1 -> Sum/2

== system Ackerman Model For Simulation/Left Motor/FOC1/ABC to qd ==
  abc : Inport
  wt : Inport  Port=2
  Demux : Demux  Outputs=3
  Terminator : Terminator
  Unit Delay : UnitDelay  SampleTime=-1  HasFrameUpgradeWarning=on
  Unit Delay1 : UnitDelay  SampleTime=-1  HasFrameUpgradeWarning=on
  abc to dq0 : powerlib_meascontrol/Transformations/abc to dq0  Alignment=90 degrees behind phase A axis
  id : Outport
  iq : Outport  Port=2
  wires:
  abc/1 -> abc to dq0/1
  Unit Delay1/1 -> id/1
  wt/1 -> abc to dq0/2
  Unit Delay/1 -> iq/1
  Demux/2 -> Unit Delay1/1
  abc to dq0/1 -> Demux/1
  Demux/3 -> Terminator/1
  Demux/1 -> Unit Delay/1

== system Ackerman Model For Simulation/Left Motor/FOC1/Phir calculation ==
  id : Inport
  Transfer Fcn : TransferFcn  Numerator=[Lm]  Denominator=[Tr 1]
  Phir : Outport
  wires:
  id/1 -> Transfer Fcn/1
  Transfer Fcn/1 -> Phir/1

== system Ackerman Model For Simulation/Left Motor/FOC1/SVPWM ==
  In1 : Inport
  In2 : Inport  Port=2
  Constant1 : Constant  Value=0
  Demux1 : Demux  Outputs=3
  Mux2 : Mux  Inputs=3
  SVPWM Generator (2-Level) : powerlib_meascontrol/Pulse & Signal Generators/SVPWM Generator (2-Level)  InputType=alpha-beta components  SwitchingPattern=Pattern #1  Fc=5000  ParUref=[0.8 -30 50]  Ts=0
      settings: SourceProductBaseCode=PS
  Terminator1 : Terminator
  dq0 to Alpha-Beta-Zero : powerlib_meascontrol/Transformations/dq0 to Alpha-Beta-Zero  Alignment=90 degrees behind phase A axis
      settings: SourceProductBaseCode=PS
  P : Outport
  wires:
  Demux1/1 -> SVPWM Generator (2-Level)/1
  Constant1/1 -> Mux2/3
  dq0 to Alpha-Beta-Zero/1 -> Demux1/1
  [ThetaL] -> dq0 to Alpha-Beta-Zero/2
  In2/1 -> Mux2/2
  SVPWM Generator (2-Level)/1 -> P/1
  In1/1 -> Mux2/1
  Mux2/1 -> dq0 to Alpha-Beta-Zero/1
  Demux1/3 -> Terminator1/1
  Demux1/2 -> SVPWM Generator (2-Level)/2

== system Ackerman Model For Simulation/Left Motor/FOC1/Theta calulation ==
  Phir : Inport
  iq : Inport  Port=2
  wm : Inport  Port=3
  Add : Sum
  Discrete-Time Integrator : DiscreteIntegrator  SampleTime=Ts  ICPrevOutput=DiscIntNeverNeededParam  ICPrevScaledInput=DiscIntNeverNeededParam
  Fcn1 : Fcn  Expr=Lm*u(2)/(u(1)*Tr+1e-3)
  Gain1 : Gain  Gain=P/2
  Mux1 : Mux  Inputs=2
  Scope : Scope  NumInputPorts=2
  theta : Outport
  wires:
  Discrete-Time Integrator/1 -> theta/1, Scope/1
  iq/1 -> Mux1/2
  wm/1 -> Gain1/1
  Add/1 -> Discrete-Time Integrator/1, Scope/2
  Mux1/1 -> Fcn1/1
  Fcn1/1 -> Add/1
  Phir/1 -> Mux1/1
  Gain1/1 -> Add/2

== system Ackerman Model For Simulation/Left Motor/FOC1/Vd ==
  Phir* : Inport
  id : Inport  Port=2
  Current PI : pid_lib/PID Controller  Controller=PI  Form=Parallel  TimeDomain=Discrete-time  UseExternalTs=off  SampleTime=Ts  IntegratorMethod=Forward Euler  FilterMethod=Forward Euler  ControllerParametersSource=internal  P=Kp  I=Ki  D=0  UseFilter=on  N=100  TunerSelectOption=Transfer Function Based (PID Tuner App)  InitialConditionSource=internal  InitialConditionForIntegrator=0  InitialConditionForFilter=0  DifferentiatorICPrevScaledInput=0  ExternalReset=none  TrackingMode=off  Kt=1  LimitOutput=on  SatLimitsSource=internal  UpperSaturationLimit=VDC  LowerSaturationLimit=-VDC/2  LinearizeAsGain=off  AntiWindupMode=clamping  Kb=1  POutMin=[]  POutMax=[]  IOutMin=[]  IOutMax=[]  DOutMin=[]  DOutMax=[]  NOutMin=[]  NOutMax=[]  SumOutMin=[]  SumOutMax=[]  SaturationOutMin=[]  SaturationOutMax=[]  PParamMin=[]  PParamMax=[]  IParamMin=[]  IParamMax=[]  DParamMin=[]  DParamMax=[]  NParamMin=[]  NParamMax=[]  KbParamMin=[]  KbParamMax=[]  KtParamMin=[]  KtParamMax=[]  KbOutMin=[]  KbOutMax=[]  KtOutMin=[]  KtOutMax=[]  IntegratorOutMin=[]  IntegratorOutMax=[]  FilterOutMin=[]  FilterOutMax=[]  SumI1OutMin=[]  SumI1OutMax=[]  SumI2OutMin=[]  SumI2OutMax=[]  SumI3OutMin=[]  SumI3OutMax=[]  SumI4OutMin=[]  SumI4OutMax=[]  SumDOutMin=[]  SumDOutMax=[]  DifferentiatorOutMin=[]  DifferentiatorOutMax=[]  FilterDiffOutCoefMin=[]  FilterDiffOutCoefMax=[]  ReciprocalOutMin=[]  ReciprocalOutMax=[]  SumDenOutMin=[]  SumDenOutMax=[]  SumNumOutMin=[]  SumNumOutMax=[]  DivideOutMin=[]  DivideOutMax=[]  UdiffTsProdOutMin=[]  UdiffTsProdOutMax=[]  NTsProdOutMin=[]  NTsProdOutMax=[]  UintegralTsProdOutMin=[]  UintegralTsProdOutMax=[]  UngainTsProdOutMin=[]  UngainTsProdOutMax=[]  IntegratorContinuousStateAttributes=''  IntegratorStateMustResolveToSignalObject=off  IntegratorRTWStateStorageClass=Auto  FilterContinuousStateAttributes=''  FilterStateMustResolveToSignalObject=off  FilterRTWStateStorageClass=Auto  ParallelPVariant=InternalParameters  IdealPVariant=Disabled  IVariant=InternalParameters  DVariant=Disabled  IntegratorVariant=Discrete  SatVariant=Enabled  AWVariant=DiscClampingParallel  PCopyVariant=Disabled  TRVariant=Disabled  FdbkBlocksVariant=Forward  IdealPFdbkVariant=Disabled  SatFdbkVariant=Disabled  DerivativeFilterVariant=Disabled  NVariant=Disabled  NCopyVariant=Disabled_SignalSpec  FilterICVariant=Disabled  IntegratorICVariant=InternalICs  ExternalResetVariant=Disabled  TRSumVariant=Passthrough  SumFdbkVariant=Disabled  SumVariant=Sum_PI  TsampFilterVariant=InternalTs  TsampNgainVariant=Passthrough  TsampIntegralVariant=Passthrough  ExternalSaturationOutDataTypeStr=Inherit: Same as second input
  Gain : Gain  Gain=1/Lm
  Scope : Scope
  Sum2 : Sum  Inputs=|+-
  Vd : Outport
  tag scope: IdrefL=global
  wires:
  Current PI/1 -> Vd/1
  Sum2/1 -> Current PI/1
  id/1 -> Sum2/2
  Phir*/1 -> Gain/1
  Gain/1 -> Sum2/1, Scope/1, [IdrefL]
